simulink model "ReglarePI_cascada"  (R2024b)
settings: Solver=VariableStepAuto  StartTime=0.0  StopTime=1000  RelTol=1e-3
values from neighbouring files (symbols this model uses):
  A = 332.5    [date_indrumator.m]
  C = 9    [date_indrumator.m]
  h0 = 10.5    [date_indrumator.m]
  href = 13    [date_indrumator.m]
  k = 0.035    [date_indrumator.m]    (also in proiect.m)
  k1 = 0.6241    [date_indrumator.m]    (also in proiect.m = 0.624)
  k11 = k2^2 + 4*(k - k3)*k1    (= 0.08909684)    [date_indrumator.m]    (also in proiect.m = 0.08885985)
  k12 = 8*(k-k3)    (= 0.2848)    [date_indrumator.m]    (also in proiect.m)
  k13 = 2*(k-k3)    (= 0.0712)    [date_indrumator.m]    (also in proiect.m)
  k2 = -0.015    [date_indrumator.m]    (also in proiect.m = -0.0015)
  k3 = -0.0006    [date_indrumator.m]    (also in proiect.m)
  keta = 8*(10^-5)    (= 8e-05)    [date_indrumator.m]    (also in proiect.m)
  q0 = 29.18    [date_indrumator.m]
  q_cascada = 34.42    [date_indrumator.m]
undefined symbols (not defined in the file or in its folder): Krpe, Krpi
libraries: slpidlib x3
settings Model: Creator=Ruxandra  LastModifiedBy=Ruxandra

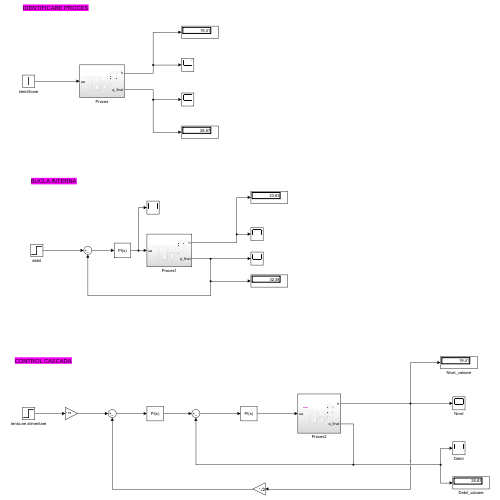
[thumbnail: Simulink's stored preview of the top-level diagram]
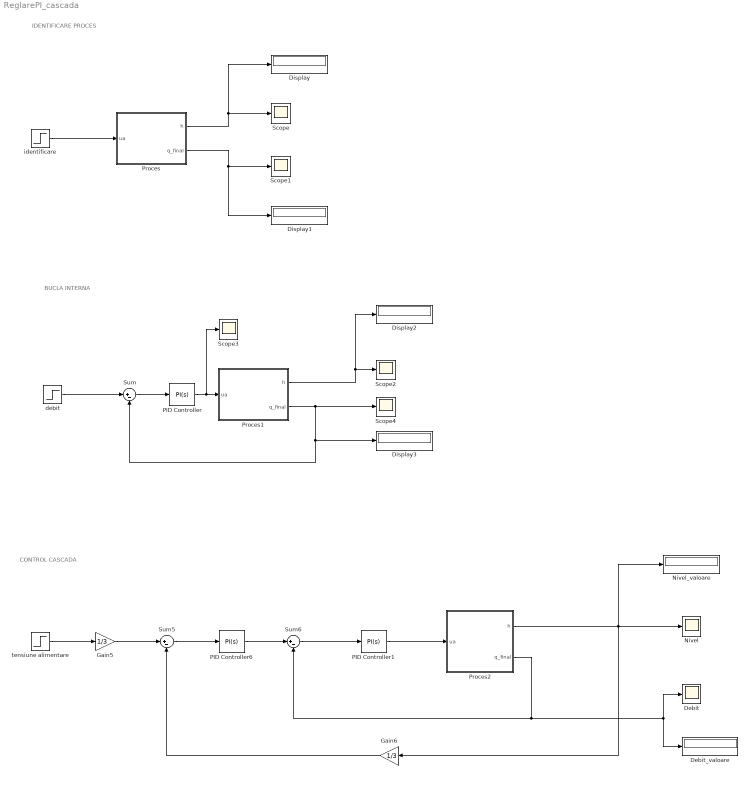
== system ReglarePI_cascada ==
  note: IDENTIFICARE PROCES
  note: BUCLA INTERNA
  note: CONTROL CASCADA
  Debit : Scope
  Debit_valoare : Display
  Display{,1..3} (4 alike) : Display
  Gain5 : Gain  Gain=1/3
  Gain6 : Gain  Gain=1/3
  Nivel : Scope
  Nivel_valoare : Display
  PID Controller : slpidlib/PID Controller  Controller=PI  Form=Parallel  TimeDomain=Continuous-time  UseExternalTs=off  SampleTime=-1  IntegratorMethod=Forward Euler  FilterMethod=Forward Euler  ControllerParametersSource=internal  P=Krpi  I=Krpi/Trpi  UseKiTs=off  D=0  UseExternalDerivativeSource=off  N=100  UseFilter=on  TunerSelectOption=Transfer Function Based (PID Tuner App)  InitialConditionSource=internal  InitialConditionForIntegrator=5  InitialConditionForFilter=0  DifferentiatorICPrevScaledInput=0  ExternalReset=none  TrackingMode=off  Kt=1  LimitOutput=off  SatLimitsSource=internal  UpperSaturationLimit=inf  LowerSaturationLimit=-inf  LinearizeAsGain=on  AntiWindupMode=none  Kb=1  LimitIntegrator=off  UpperIntegratorSaturationLimit=inf  LowerIntegratorSaturationLimit=-inf  POutMin=[]  POutMax=[]  IOutMin=[]  IOutMax=[]  DOutMin=[]  DOutMax=[]  NOutMin=[]  NOutMax=[]  SumOutMin=[]  SumOutMax=[]  SaturationOutMin=[]  SaturationOutMax=[]  PParamMin=[]  PParamMax=[]  IParamMin=[]  IParamMax=[]  DParamMin=[]  DParamMax=[]  NParamMin=[]  NParamMax=[]  KbParamMin=[]  KbParamMax=[]  KtParamMin=[]  KtParamMax=[]  KbOutMin=[]  KbOutMax=[]  KtOutMin=[]  KtOutMax=[]  IntegratorOutMin=[]  IntegratorOutMax=[]  FilterOutMin=[]  FilterOutMax=[]  SumI1OutMin=[]  SumI1OutMax=[]  SumI2OutMin=[]  SumI2OutMax=[]  SumI3OutMin=[]  SumI3OutMax=[]  SumI4OutMin=[]  SumI4OutMax=[]  SumDOutMin=[]  SumDOutMax=[]  DifferentiatorOutMin=[]  DifferentiatorOutMax=[]  FilterDiffOutCoefMin=[]  FilterDiffOutCoefMax=[]  ReciprocalOutMin=[]  ReciprocalOutMax=[]  SumDenOutMin=[]  SumDenOutMax=[]  SumNumOutMin=[]  SumNumOutMax=[]  DivideOutMin=[]  DivideOutMax=[]  UdiffTsProdOutMin=[]  UdiffTsProdOutMax=[]  NTsProdOutMin=[]  NTsProdOutMax=[]  UintegralTsProdOutMin=[]  UintegralTsProdOutMax=[]  UngainTsProdOutMin=[]  UngainTsProdOutMax=[]  ClampingZeroOutDataTypeStr=Inherit: Inherit via back propagation  ClampingZeroOutMin=[]  ClampingZeroOutMax=[]  FilterDenConstantOutDataTypeStr=Inherit: Inherit via back propagation  FilterDenConstantOutMin=[]  FilterDenConstantOutMax=[]  PCopyOutDataTypeStr=Inherit: Inherit via back propagation  PCopyOutMin=[]  PCopyOutMax=[]  NCopyOutDataTypeStr=Inherit: Inherit via back propagation  NCopyOutMin=[]  NCopyOutMax=[]  IntegratorContinuousStateAttributes=''  IntegratorStateMustResolveToSignalObject=off  IntegratorRTWStateStorageClass=Auto  FilterContinuousStateAttributes=''  FilterStateMustResolveToSignalObject=off  FilterRTWStateStorageClass=Auto  ParallelPVariant=InternalParameters  IdealPVariant=Disabled  IVariant=InternalParameters  DVariant=Disabled  IntegratorVariant=Continuous  SatVariant=Disabled  AWVariant=Passthrough  PCopyVariant=Disabled  TRVariant=Disabled  FdbkBlocksVariant=Forward  IdealPFdbkVariant=Disabled  SatFdbkVariant=Disabled  DerivativeFilterVariant=Disabled  NVariant=Disabled  NCopyVariant=Disabled_SignalSpec  FilterICVariant=Disabled  IntegratorICVariant=InternalICs  ExternalResetVariant=Disabled  TRSumVariant=Passthrough  SumFdbkVariant=Disabled  SumVariant=Sum_PI  TsampFilterVariant=InternalTs  TsampNgainVariant=Passthrough  TsampIntegralVariant=Disabled_SignalSpec  ExternalSaturationOutDataTypeStr=Inherit: Same as second input  DerivativeSourceVariant=Disabled  PreIntVariant=InternalPreInt
  PID Controller1 : slpidlib/PID Controller  Controller=PI  Form=Parallel  TimeDomain=Continuous-time  UseExternalTs=off  SampleTime=-1  IntegratorMethod=Forward Euler  FilterMethod=Forward Euler  ControllerParametersSource=internal  P=Krpi  I=Krpi/Trpi  UseKiTs=off  D=0  UseExternalDerivativeSource=off  N=100  UseFilter=on  TunerSelectOption=Transfer Function Based (PID Tuner App)  InitialConditionSource=internal  InitialConditionForIntegrator=5  InitialConditionForFilter=0  DifferentiatorICPrevScaledInput=0  ExternalReset=none  TrackingMode=off  Kt=1  LimitOutput=off  SatLimitsSource=internal  UpperSaturationLimit=inf  LowerSaturationLimit=-inf  LinearizeAsGain=on  AntiWindupMode=none  Kb=1  LimitIntegrator=off  UpperIntegratorSaturationLimit=inf  LowerIntegratorSaturationLimit=-inf  POutMin=[]  POutMax=[]  IOutMin=[]  IOutMax=[]  DOutMin=[]  DOutMax=[]  NOutMin=[]  NOutMax=[]  SumOutMin=[]  SumOutMax=[]  SaturationOutMin=[]  SaturationOutMax=[]  PParamMin=[]  PParamMax=[]  IParamMin=[]  IParamMax=[]  DParamMin=[]  DParamMax=[]  NParamMin=[]  NParamMax=[]  KbParamMin=[]  KbParamMax=[]  KtParamMin=[]  KtParamMax=[]  KbOutMin=[]  KbOutMax=[]  KtOutMin=[]  KtOutMax=[]  IntegratorOutMin=[]  IntegratorOutMax=[]  FilterOutMin=[]  FilterOutMax=[]  SumI1OutMin=[]  SumI1OutMax=[]  SumI2OutMin=[]  SumI2OutMax=[]  SumI3OutMin=[]  SumI3OutMax=[]  SumI4OutMin=[]  SumI4OutMax=[]  SumDOutMin=[]  SumDOutMax=[]  DifferentiatorOutMin=[]  DifferentiatorOutMax=[]  FilterDiffOutCoefMin=[]  FilterDiffOutCoefMax=[]  ReciprocalOutMin=[]  ReciprocalOutMax=[]  SumDenOutMin=[]  SumDenOutMax=[]  SumNumOutMin=[]  SumNumOutMax=[]  DivideOutMin=[]  DivideOutMax=[]  UdiffTsProdOutMin=[]  UdiffTsProdOutMax=[]  NTsProdOutMin=[]  NTsProdOutMax=[]  UintegralTsProdOutMin=[]  UintegralTsProdOutMax=[]  UngainTsProdOutMin=[]  UngainTsProdOutMax=[]  ClampingZeroOutDataTypeStr=Inherit: Inherit via back propagation  ClampingZeroOutMin=[]  ClampingZeroOutMax=[]  FilterDenConstantOutDataTypeStr=Inherit: Inherit via back propagation  FilterDenConstantOutMin=[]  FilterDenConstantOutMax=[]  PCopyOutDataTypeStr=Inherit: Inherit via back propagation  PCopyOutMin=[]  PCopyOutMax=[]  NCopyOutDataTypeStr=Inherit: Inherit via back propagation  NCopyOutMin=[]  NCopyOutMax=[]  IntegratorContinuousStateAttributes=''  IntegratorStateMustResolveToSignalObject=off  IntegratorRTWStateStorageClass=Auto  FilterContinuousStateAttributes=''  FilterStateMustResolveToSignalObject=off  FilterRTWStateStorageClass=Auto  ParallelPVariant=InternalParameters  IdealPVariant=Disabled  IVariant=InternalParameters  DVariant=Disabled  IntegratorVariant=Continuous  SatVariant=Disabled  AWVariant=Passthrough  PCopyVariant=Disabled  TRVariant=Disabled  FdbkBlocksVariant=Forward  IdealPFdbkVariant=Disabled  SatFdbkVariant=Disabled  DerivativeFilterVariant=Disabled  NVariant=Disabled  NCopyVariant=Disabled_SignalSpec  FilterICVariant=Disabled  IntegratorICVariant=InternalICs  ExternalResetVariant=Disabled  TRSumVariant=Passthrough  SumFdbkVariant=Disabled  SumVariant=Sum_PI  TsampFilterVariant=InternalTs  TsampNgainVariant=Passthrough  TsampIntegralVariant=Disabled_SignalSpec  ExternalSaturationOutDataTypeStr=Inherit: Same as second input  DerivativeSourceVariant=Disabled  PreIntVariant=InternalPreInt
  PID Controller6 : slpidlib/PID Controller  Controller=PI  Form=Parallel  TimeDomain=Continuous-time  UseExternalTs=off  SampleTime=-1  IntegratorMethod=Forward Euler  FilterMethod=Forward Euler  ControllerParametersSource=internal  P=Krpe  I=Krpe/Trpe  UseKiTs=off  D=0  UseExternalDerivativeSource=off  N=100  UseFilter=on  TunerSelectOption=Transfer Function Based (PID Tuner App)  InitialConditionSource=internal  InitialConditionForIntegrator=q0  InitialConditionForFilter=0  DifferentiatorICPrevScaledInput=0  ExternalReset=none  TrackingMode=off  Kt=1  LimitOutput=off  SatLimitsSource=internal  UpperSaturationLimit=inf  LowerSaturationLimit=-inf  LinearizeAsGain=on  AntiWindupMode=none  Kb=1  LimitIntegrator=off  UpperIntegratorSaturationLimit=inf  LowerIntegratorSaturationLimit=-inf  POutMin=[]  POutMax=[]  IOutMin=[]  IOutMax=[]  DOutMin=[]  DOutMax=[]  NOutMin=[]  NOutMax=[]  SumOutMin=[]  SumOutMax=[]  SaturationOutMin=[]  SaturationOutMax=[]  PParamMin=[]  PParamMax=[]  IParamMin=[]  IParamMax=[]  DParamMin=[]  DParamMax=[]  NParamMin=[]  NParamMax=[]  KbParamMin=[]  KbParamMax=[]  KtParamMin=[]  KtParamMax=[]  KbOutMin=[]  KbOutMax=[]  KtOutMin=[]  KtOutMax=[]  IntegratorOutMin=[]  IntegratorOutMax=[]  FilterOutMin=[]  FilterOutMax=[]  SumI1OutMin=[]  SumI1OutMax=[]  SumI2OutMin=[]  SumI2OutMax=[]  SumI3OutMin=[]  SumI3OutMax=[]  SumI4OutMin=[]  SumI4OutMax=[]  SumDOutMin=[]  SumDOutMax=[]  DifferentiatorOutMin=[]  DifferentiatorOutMax=[]  FilterDiffOutCoefMin=[]  FilterDiffOutCoefMax=[]  ReciprocalOutMin=[]  ReciprocalOutMax=[]  SumDenOutMin=[]  SumDenOutMax=[]  SumNumOutMin=[]  SumNumOutMax=[]  DivideOutMin=[]  DivideOutMax=[]  UdiffTsProdOutMin=[]  UdiffTsProdOutMax=[]  NTsProdOutMin=[]  NTsProdOutMax=[]  UintegralTsProdOutMin=[]  UintegralTsProdOutMax=[]  UngainTsProdOutMin=[]  UngainTsProdOutMax=[]  ClampingZeroOutDataTypeStr=Inherit: Inherit via back propagation  ClampingZeroOutMin=[]  ClampingZeroOutMax=[]  FilterDenConstantOutDataTypeStr=Inherit: Inherit via back propagation  FilterDenConstantOutMin=[]  FilterDenConstantOutMax=[]  PCopyOutDataTypeStr=Inherit: Inherit via back propagation  PCopyOutMin=[]  PCopyOutMax=[]  NCopyOutDataTypeStr=Inherit: Inherit via back propagation  NCopyOutMin=[]  NCopyOutMax=[]  IntegratorContinuousStateAttributes=''  IntegratorStateMustResolveToSignalObject=off  IntegratorRTWStateStorageClass=Auto  FilterContinuousStateAttributes=''  FilterStateMustResolveToSignalObject=off  FilterRTWStateStorageClass=Auto  ParallelPVariant=InternalParameters  IdealPVariant=Disabled  IVariant=InternalParameters  DVariant=Disabled  IntegratorVariant=Continuous  SatVariant=Disabled  AWVariant=Passthrough  PCopyVariant=Disabled  TRVariant=Disabled  FdbkBlocksVariant=Forward  IdealPFdbkVariant=Disabled  SatFdbkVariant=Disabled  DerivativeFilterVariant=Disabled  NVariant=Disabled  NCopyVariant=Disabled_SignalSpec  FilterICVariant=Disabled  IntegratorICVariant=InternalICs  ExternalResetVariant=Disabled  TRSumVariant=Passthrough  SumFdbkVariant=Disabled  SumVariant=Sum_PI  TsampFilterVariant=InternalTs  TsampNgainVariant=Passthrough  TsampIntegralVariant=Disabled_SignalSpec  ExternalSaturationOutDataTypeStr=Inherit: Same as second input  DerivativeSourceVariant=Disabled  PreIntVariant=InternalPreInt
  Proces : Subsystem
  Proces1 : Subsystem
  Proces2 : Subsystem
  Scope{,1..4} (5 alike) : Scope
  Sum : Sum  Inputs=|+-
  Sum5 : Sum  Inputs=|+-
  Sum6 : Sum  Inputs=|+-
  debit : Step  Time=0  Before=q0  After=q_cascada  SampleTime=0
  identificare : Step  Time=0  Before=5  After=5.5  SampleTime=0
  tensiune alimentare : Step  Time=0  After=href  SampleTime=0
  wires:
  identificare/1 -> Proces/1(ua)
  Proces/1(h) -> Display/1, Scope/1
  Proces/2(q_final) -> Display1/1, Scope1/1
  debit/1 -> Sum/1
  Sum/1 -> PID Controller/1
  Proces1/1(h) -> Display2/1, Scope2/1
  PID Controller/1 -> Scope3/1, Proces1/1(ua)
  Proces1/2(q_final) -> Display3/1, Sum/2, Scope4/1
  Sum5/1 -> PID Controller6/1
  Sum6/1 -> PID Controller1/1
  Proces2/1(h) -> Nivel_valoare/1, Gain6/1, Nivel/1
  PID Controller1/1 -> Proces2/1(ua)
  PID Controller6/1 -> Sum6/1
  Proces2/2(q_final) -> Sum6/2, Debit/1, Debit_valoare/1
  Gain5/1 -> Sum5/1
  Gain6/1 -> Sum5/2
  tensiune alimentare/1 -> Gain5/1

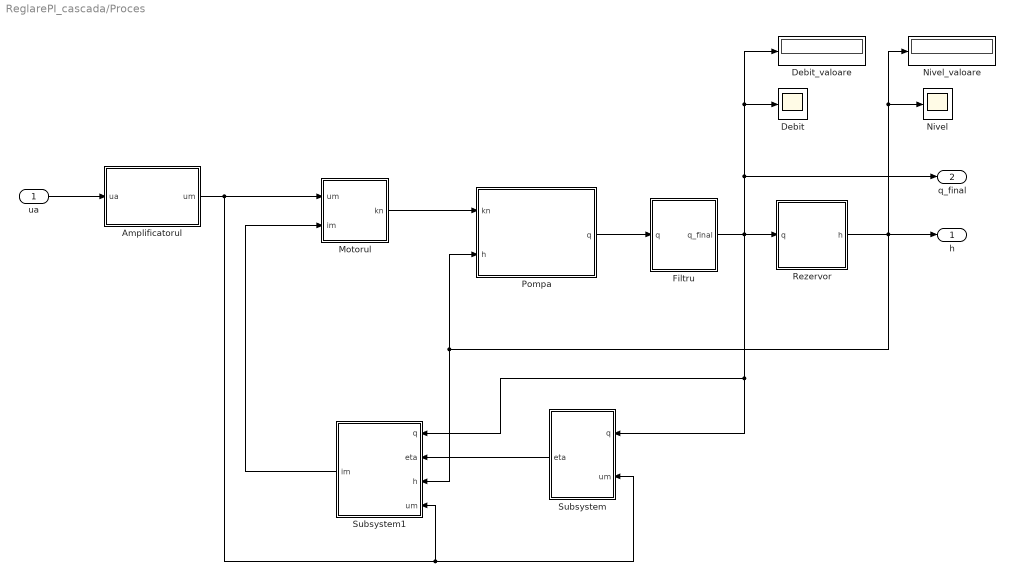
== system ReglarePI_cascada/Proces ==
  ua : Inport
  Amplificatorul : Subsystem
  Debit : Scope
  Debit_valoare : Display
  Filtru : Subsystem
  Motorul : Subsystem
  Nivel : Scope
  Nivel_valoare : Display
  Pompa : Subsystem
  Rezervor : Subsystem
  Subsystem : Subsystem
  Subsystem1 : Subsystem
  h : Outport
  q_final : Outport  Port=2
  wires:
  Subsystem/1(eta) -> Subsystem1/2(eta)
  Filtru/1(q_final) -> q_final/1, Debit_valoare/1, Debit/1, Subsystem1/1(q), Subsystem/1(q), Rezervor/1(q)
  ua/1 -> Amplificatorul/1(ua)
  Rezervor/1(h) -> h/1, Pompa/2(h), Subsystem1/3(h), Nivel_valoare/1, Nivel/1
  Pompa/1(q) -> Filtru/1(q)
  Motorul/1("kn ") -> Pompa/1(kn)
  Amplificatorul/1(um) -> Motorul/1(um), Subsystem1/4(um), Subsystem/2(um)
  Subsystem1/1(im) -> Motorul/2(im)

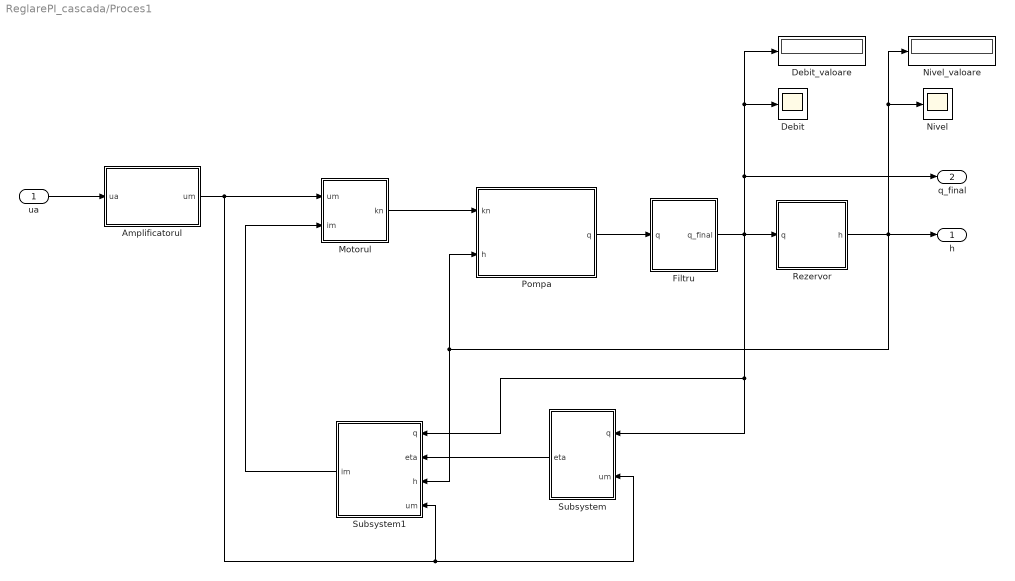
== system ReglarePI_cascada/Proces1 ==
  ua : Inport
  Amplificatorul : Subsystem
  Debit : Scope
  Debit_valoare : Display
  Filtru : Subsystem
  Motorul : Subsystem
  Nivel : Scope
  Nivel_valoare : Display
  Pompa : Subsystem
  Rezervor : Subsystem
  Subsystem : Subsystem
  Subsystem1 : Subsystem
  h : Outport
  q_final : Outport  Port=2
  wires:
  Subsystem1/1(im) -> Motorul/2(im)
  Amplificatorul/1(um) -> Subsystem/2(um), Subsystem1/4(um), Motorul/1(um)
  Motorul/1("kn ") -> Pompa/1(kn)
  Pompa/1(q) -> Filtru/1(q)
  Rezervor/1(h) -> Nivel/1, Nivel_valoare/1, Subsystem1/3(h), Pompa/2(h), h/1
  ua/1 -> Amplificatorul/1(ua)
  Filtru/1(q_final) -> Rezervor/1(q), Subsystem/1(q), Subsystem1/1(q), Debit/1, Debit_valoare/1, q_final/1
  Subsystem/1(eta) -> Subsystem1/2(eta)

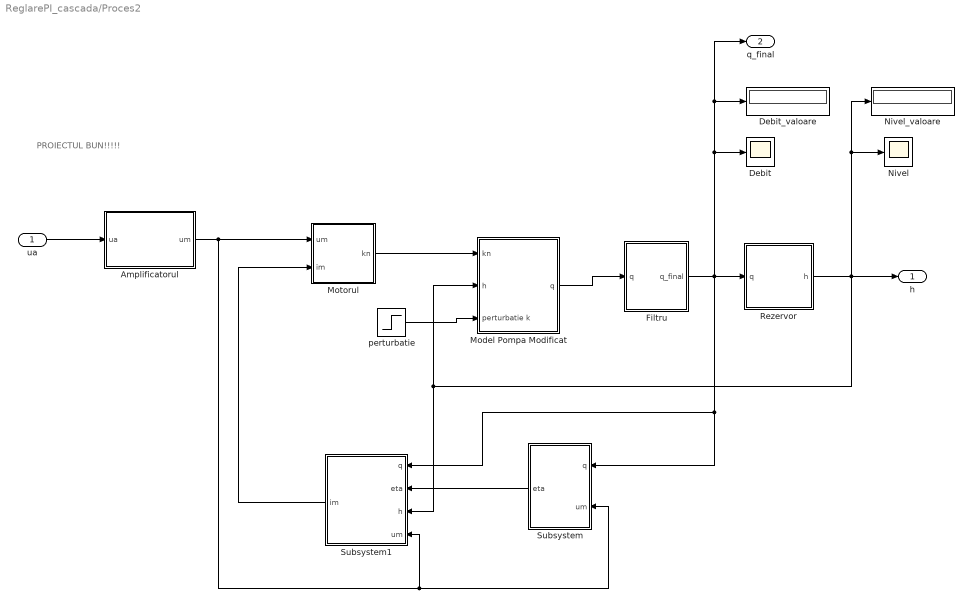
== system ReglarePI_cascada/Proces2 ==
  note: PROIECTUL BUN!!!!!
  ua : Inport
  Amplificatorul : Subsystem
  Debit : Scope
  Debit_valoare : Display
  Filtru : Subsystem
  Model Pompa Modificat : Subsystem
  Motorul : Subsystem
  Nivel : Scope
  Nivel_valoare : Display
  Rezervor : Subsystem
  Subsystem : Subsystem
  Subsystem1 : Subsystem
  perturbatie : Step  Time=250  After=0.3*k  SampleTime=0
  h : Outport
  q_final : Outport  Port=2
  wires:
  ua/1 -> Amplificatorul/1(ua)
  Motorul/1("kn ") -> Model Pompa Modificat/1(kn)
  Amplificatorul/1(um) -> Motorul/1(um), Subsystem1/4(um), Subsystem/2(um)
  Subsystem/1(eta) -> Subsystem1/2(eta)
  Rezervor/1(h) -> h/1, Model Pompa Modificat/2(h), Subsystem1/3(h), Nivel_valoare/1, Nivel/1
  Model Pompa Modificat/1(q) -> Filtru/1(q)
  Subsystem1/1(im) -> Motorul/2(im)
  Filtru/1(q_final) -> q_final/1, Debit_valoare/1, Debit/1, Subsystem1/1(q), Subsystem/1(q), Rezervor/1(q)
  perturbatie/1 -> Model Pompa Modificat/3(perturbatie k)

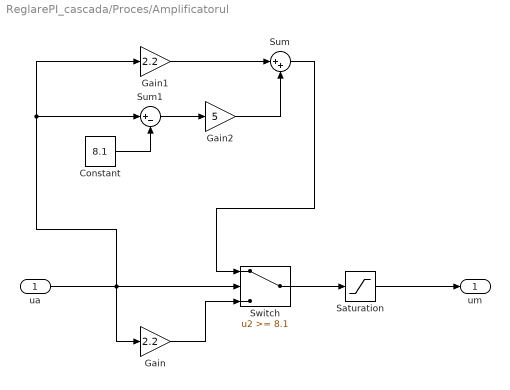
== system ReglarePI_cascada/Proces/Amplificatorul ==
  ua : Inport
  Constant : Constant  Value=8.1
  Gain : Gain  Gain=2.2
  Gain1 : Gain  Gain=2.2
  Gain2 : Gain  Gain=5
  Saturation : Saturate  UpperLimit=22  LowerLimit=0
  Sum : Sum  Inputs=|++
  Sum1 : Sum  Inputs=|+-
  Switch : Switch  Threshold=8.1  RndMeth=Nearest  SaturateOnIntegerOverflow=off  InputSameDT=off
  um : Outport
  wires:
  Gain/1 -> Switch/3
  Gain1/1 -> Sum/1
  Sum1/1 -> Gain2/1
  ua/1 -> Gain/1, Sum1/1, Gain1/1, Switch/2
  Saturation/1 -> um/1
  Constant/1 -> Sum1/2
  Sum/1 -> Switch/1
  Switch/1 -> Saturation/1
  Gain2/1 -> Sum/2

== system ReglarePI_cascada/Proces/Filtru ==
  q : Inport
  Integrator : Integrator  InitialCondition=q0
  Sum : Sum  Inputs=|+-
  q_final : Outport
  wires:
  Integrator/1 -> q_final/1, Sum/2
  q/1 -> Sum/1
  Sum/1 -> Integrator/1

== system ReglarePI_cascada/Proces/Motorul ==
  note: im se poate obtine in functie de nivelul din rezervor, debitul si randamentul pompei.
  um : Inport
  im : Inport  Port=2
  Add : Sum  Inputs=+-
  Rm : Gain  Gain=3
  "kn " : Outport
  wires:
  Rm/1 -> Add/2
  Add/1 -> "kn "/1
  um/1 -> Add/1
  im/1 -> Rm/1

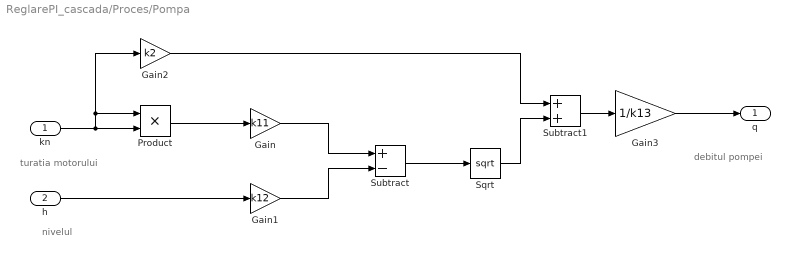
== system ReglarePI_cascada/Proces/Pompa ==
  note: nivelul
  note: turatia motorului
  note: debitul pompei
  kn : Inport
  h : Inport  Port=2
  Gain : Gain  Gain=k11
  Gain1 : Gain  Gain=k12
  Gain2 : Gain  Gain=k2
  Gain3 : Gain  Gain=1/k13
  Product : Product
  Sqrt : Sqrt
  Subtract : Sum  Inputs=+-
  Subtract1 : Sum
  q : Outport
  wires:
  Gain2/1 -> Subtract1/1
  kn/1 -> Product/1, Gain2/1, Product/2
  Gain3/1 -> q/1
  Product/1 -> Gain/1
  Gain1/1 -> Subtract/2
  Subtract/1 -> Sqrt/1
  h/1 -> Gain1/1
  Sqrt/1 -> Subtract1/2
  Gain/1 -> Subtract/1
  Subtract1/1 -> Gain3/1

== system ReglarePI_cascada/Proces/Rezervor ==
  q : Inport
  Fcn : Fcn  Expr=sqrt(u)*C
  Gain : Gain  Gain=1/A
  Integrator : Integrator  InitialCondition=h0
  Sum : Sum  Inputs=|+-
  h : Outport
  wires:
  q/1 -> Sum/1
  Gain/1 -> Integrator/1
  Sum/1 -> Gain/1
  Integrator/1 -> Fcn/1, h/1
  Fcn/1 -> Sum/2

== system ReglarePI_cascada/Proces/Subsystem ==
  note: randamentul pompei
  q : Inport
  um : Inport  Port=2
  Gain : Gain  Gain=keta
  Product : Product
  eta : Outport
  wires:
  q/1 -> Product/1
  um/1 -> Gain/1
  Gain/1 -> Product/2
  Product/1 -> eta/1

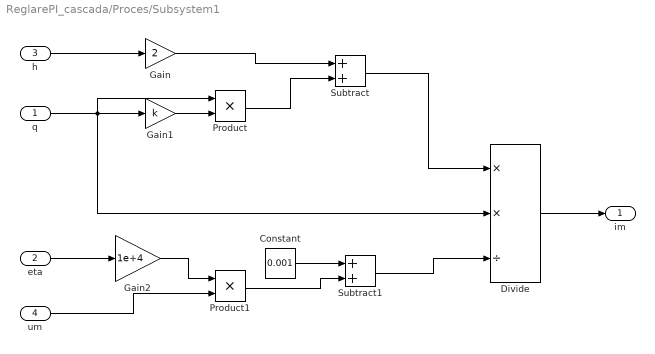
== system ReglarePI_cascada/Proces/Subsystem1 ==
  q : Inport
  eta : Inport  Port=2
  h : Inport  Port=3
  um : Inport  Port=4
  Constant : Constant  Value=0.001
  Divide : Product  Inputs=**/
  Gain : Gain  Gain=2
  Gain1 : Gain  Gain=k
  Gain2 : Gain  Gain=1e+4
  Product : Product
  Product1 : Product
  Subtract : Sum
  Subtract1 : Sum
  im : Outport
  wires:
  Subtract1/1 -> Divide/3
  Gain2/1 -> Product1/1
  h/1 -> Gain/1
  Subtract/1 -> Divide/1
  Product1/1 -> Subtract1/2
  eta/1 -> Gain2/1
  Gain1/1 -> Product/2
  um/1 -> Product1/2
  Constant/1 -> Subtract1/1
  Gain/1 -> Subtract/1
  Product/1 -> Subtract/2
  q/1 -> Divide/2, Gain1/1, Product/1
  Divide/1 -> im/1

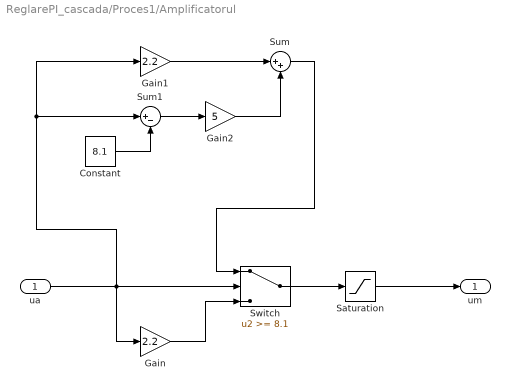
== system ReglarePI_cascada/Proces1/Amplificatorul ==
  ua : Inport
  Constant : Constant  Value=8.1
  Gain : Gain  Gain=2.2
  Gain1 : Gain  Gain=2.2
  Gain2 : Gain  Gain=5
  Saturation : Saturate  UpperLimit=22  LowerLimit=0
  Sum : Sum  Inputs=|++
  Sum1 : Sum  Inputs=|+-
  Switch : Switch  Threshold=8.1  RndMeth=Nearest  SaturateOnIntegerOverflow=off  InputSameDT=off
  um : Outport
  wires:
  Gain2/1 -> Sum/2
  Switch/1 -> Saturation/1
  Sum/1 -> Switch/1
  Constant/1 -> Sum1/2
  Saturation/1 -> um/1
  ua/1 -> Switch/2, Gain1/1, Sum1/1, Gain/1
  Sum1/1 -> Gain2/1
  Gain1/1 -> Sum/1
  Gain/1 -> Switch/3

== system ReglarePI_cascada/Proces1/Filtru ==
  q : Inport
  Integrator : Integrator  InitialCondition=q0
  Sum : Sum  Inputs=|+-
  q_final : Outport
  wires:
  Sum/1 -> Integrator/1
  q/1 -> Sum/1
  Integrator/1 -> Sum/2, q_final/1

== system ReglarePI_cascada/Proces1/Motorul ==
  note: im se poate obtine in functie de nivelul din rezervor, debitul si randamentul pompei.
  um : Inport
  im : Inport  Port=2
  Add : Sum  Inputs=+-
  Rm : Gain  Gain=3
  "kn " : Outport
  wires:
  im/1 -> Rm/1
  um/1 -> Add/1
  Add/1 -> "kn "/1
  Rm/1 -> Add/2

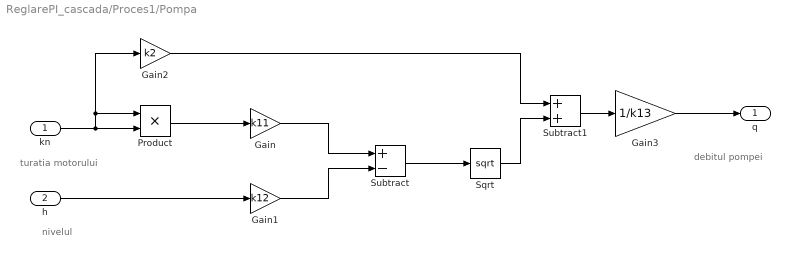
== system ReglarePI_cascada/Proces1/Pompa ==
  note: debitul pompei
  note: turatia motorului
  note: nivelul
  kn : Inport
  h : Inport  Port=2
  Gain : Gain  Gain=k11
  Gain1 : Gain  Gain=k12
  Gain2 : Gain  Gain=k2
  Gain3 : Gain  Gain=1/k13
  Product : Product
  Sqrt : Sqrt
  Subtract : Sum  Inputs=+-
  Subtract1 : Sum
  q : Outport
  wires:
  Subtract1/1 -> Gain3/1
  Gain/1 -> Subtract/1
  Sqrt/1 -> Subtract1/2
  h/1 -> Gain1/1
  Subtract/1 -> Sqrt/1
  Gain1/1 -> Subtract/2
  Product/1 -> Gain/1
  Gain3/1 -> q/1
  kn/1 -> Product/2, Gain2/1, Product/1
  Gain2/1 -> Subtract1/1

== system ReglarePI_cascada/Proces1/Rezervor ==
  q : Inport
  Fcn : Fcn  Expr=sqrt(u)*C
  Gain : Gain  Gain=1/A
  Integrator : Integrator  InitialCondition=h0
  Sum : Sum  Inputs=|+-
  h : Outport
  wires:
  Fcn/1 -> Sum/2
  Integrator/1 -> h/1, Fcn/1
  Sum/1 -> Gain/1
  Gain/1 -> Integrator/1
  q/1 -> Sum/1

== system ReglarePI_cascada/Proces1/Subsystem ==
  note: randamentul pompei
  q : Inport
  um : Inport  Port=2
  Gain : Gain  Gain=keta
  Product : Product
  eta : Outport
  wires:
  Product/1 -> eta/1
  Gain/1 -> Product/2
  um/1 -> Gain/1
  q/1 -> Product/1

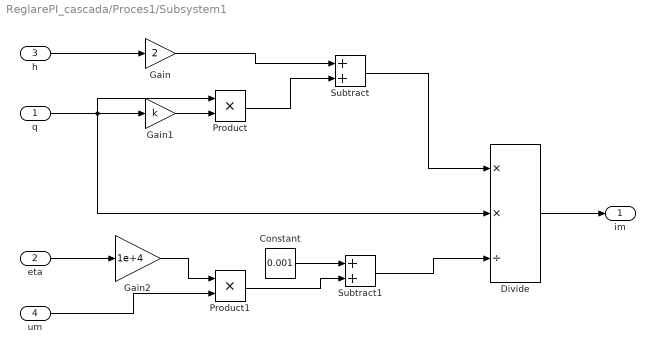
== system ReglarePI_cascada/Proces1/Subsystem1 ==
  q : Inport
  eta : Inport  Port=2
  h : Inport  Port=3
  um : Inport  Port=4
  Constant : Constant  Value=0.001
  Divide : Product  Inputs=**/
  Gain : Gain  Gain=2
  Gain1 : Gain  Gain=k
  Gain2 : Gain  Gain=1e+4
  Product : Product
  Product1 : Product
  Subtract : Sum
  Subtract1 : Sum
  im : Outport
  wires:
  Divide/1 -> im/1
  q/1 -> Product/1, Gain1/1, Divide/2
  Product/1 -> Subtract/2
  Gain/1 -> Subtract/1
  Constant/1 -> Subtract1/1
  um/1 -> Product1/2
  Gain1/1 -> Product/2
  eta/1 -> Gain2/1
  Product1/1 -> Subtract1/2
  Subtract/1 -> Divide/1
  h/1 -> Gain/1
  Gain2/1 -> Product1/1
  Subtract1/1 -> Divide/3

== system ReglarePI_cascada/Proces2/Amplificatorul ==
  ua : Inport
  Constant : Constant  Value=8.1
  Gain : Gain  Gain=2.2
  Gain1 : Gain  Gain=2.2
  Gain2 : Gain  Gain=5
  Saturation : Saturate  UpperLimit=22  LowerLimit=0
  Sum : Sum  Inputs=|++
  Sum1 : Sum  Inputs=|+-
  Switch : Switch  Threshold=8.1  RndMeth=Nearest  SaturateOnIntegerOverflow=off  InputSameDT=off
  um : Outport
  wires:
  Gain/1 -> Switch/3
  Gain1/1 -> Sum/1
  Sum1/1 -> Gain2/1
  ua/1 -> Gain/1, Sum1/1, Gain1/1, Switch/2
  Saturation/1 -> um/1
  Constant/1 -> Sum1/2
  Sum/1 -> Switch/1
  Switch/1 -> Saturation/1
  Gain2/1 -> Sum/2

== system ReglarePI_cascada/Proces2/Filtru ==
  q : Inport
  Integrator : Integrator  InitialCondition=q0
  Sum : Sum  Inputs=|+-
  q_final : Outport
  wires:
  Integrator/1 -> q_final/1, Sum/2
  q/1 -> Sum/1
  Sum/1 -> Integrator/1

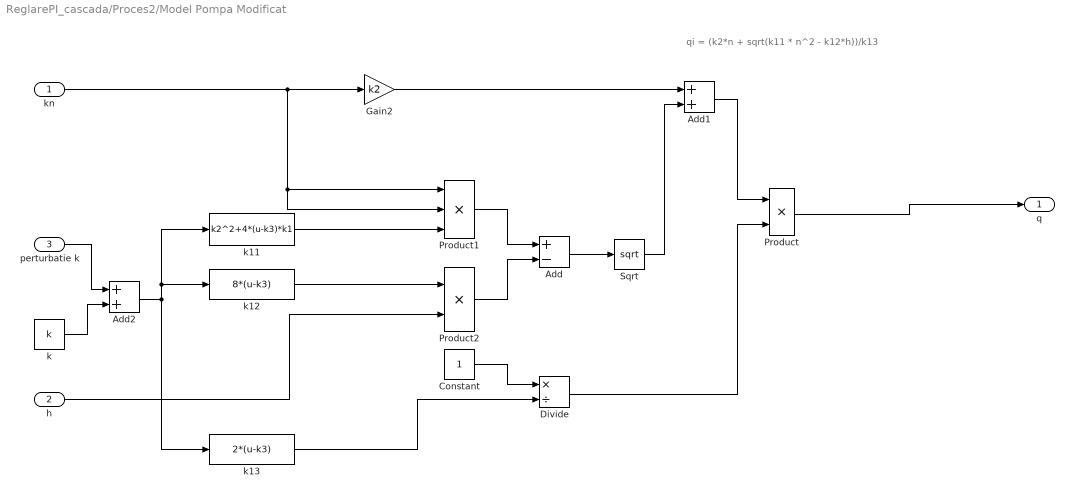
== system ReglarePI_cascada/Proces2/Model Pompa Modificat ==
  note: qi = (k2*n + sqrt(k11 * n^2 - k12*h))/k13
  kn : Inport
  h : Inport  Port=2
  perturbatie k : Inport  Port=3
  Add : Sum  Inputs=+-
  Add1 : Sum
  Add2 : Sum
  Constant : Constant
  Divide : Product  Inputs=*/
  Gain2 : Gain  Gain=k2
  Product : Product
  Product1 : Product  Inputs=3
  Product2 : Product
  Sqrt : Sqrt
  k : Constant  Value=k
  k11 : Fcn  Expr=k2^2+4*(u-k3)*k1
  k12 : Fcn  Expr=8*(u-k3)
  k13 : Fcn  Expr=2*(u-k3)
  q : Outport
  wires:
  h/1 -> Product2/2
  Sqrt/1 -> Add1/2
  Add1/1 -> Product/1
  Add/1 -> Sqrt/1
  Gain2/1 -> Add1/1
  kn/1 -> Product1/2, Product1/1, Gain2/1
  Product1/1 -> Add/1
  Product2/1 -> Add/2
  perturbatie k/1 -> Add2/1
  k/1 -> Add2/2
  Add2/1 -> k12/1, k11/1, k13/1
  k11/1 -> Product1/3
  k12/1 -> Product2/1
  Constant/1 -> Divide/1
  k13/1 -> Divide/2
  Divide/1 -> Product/2
  Product/1 -> q/1

== system ReglarePI_cascada/Proces2/Motorul ==
  note: im se poate obtine in functie de nivelul din rezervor, debitul si randamentul pompei.
  um : Inport
  im : Inport  Port=2
  Add : Sum  Inputs=+-
  Rm : Gain  Gain=3
  "kn " : Outport
  wires:
  Rm/1 -> Add/2
  Add/1 -> "kn "/1
  um/1 -> Add/1
  im/1 -> Rm/1

== system ReglarePI_cascada/Proces2/Rezervor ==
  q : Inport
  Fcn : Fcn  Expr=sqrt(u)*C
  Gain : Gain  Gain=1/A
  Integrator : Integrator  InitialCondition=h0
  Sum : Sum  Inputs=|+-
  h : Outport
  wires:
  q/1 -> Sum/1
  Gain/1 -> Integrator/1
  Sum/1 -> Gain/1
  Integrator/1 -> Fcn/1, h/1
  Fcn/1 -> Sum/2

== system ReglarePI_cascada/Proces2/Subsystem ==
  note: randamentul pompei
  q : Inport
  um : Inport  Port=2
  Gain : Gain  Gain=keta
  Product : Product
  eta : Outport
  wires:
  q/1 -> Product/1
  um/1 -> Gain/1
  Gain/1 -> Product/2
  Product/1 -> eta/1

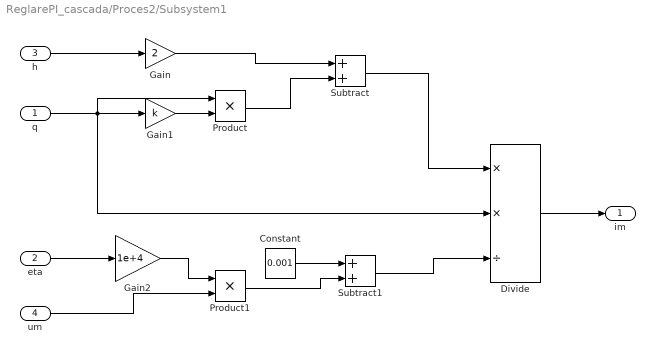
== system ReglarePI_cascada/Proces2/Subsystem1 ==
  q : Inport
  eta : Inport  Port=2
  h : Inport  Port=3
  um : Inport  Port=4
  Constant : Constant  Value=0.001
  Divide : Product  Inputs=**/
  Gain : Gain  Gain=2
  Gain1 : Gain  Gain=k
  Gain2 : Gain  Gain=1e+4
  Product : Product
  Product1 : Product
  Subtract : Sum
  Subtract1 : Sum
  im : Outport
  wires:
  Subtract1/1 -> Divide/3
  Gain2/1 -> Product1/1
  h/1 -> Gain/1
  Subtract/1 -> Divide/1
  Product1/1 -> Subtract1/2
  eta/1 -> Gain2/1
  Gain1/1 -> Product/2
  um/1 -> Product1/2
  Constant/1 -> Subtract1/1
  Gain/1 -> Subtract/1
  Product/1 -> Subtract/2
  q/1 -> Divide/2, Gain1/1, Product/1
  Divide/1 -> im/1
